simulink library "MotorModelDiscreteTfSL"  (R2016b)
settings: Solver=VariableStepAuto  StartTime=0.0  StopTime=10.0  RelTol=1e-3
undefined symbols (not defined in the file): Z0, Z1, Z2, Znom
settings Model: Creator=oelkawok  LastModifiedBy=oelkawok

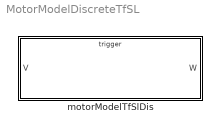
== system MotorModelDiscreteTfSL ==
  motorModelTfSlDis : Subsystem

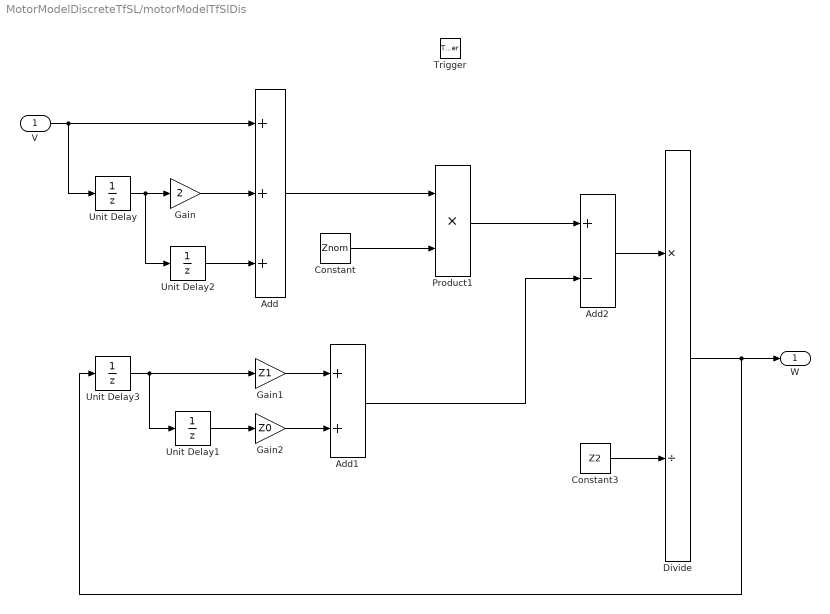
== system MotorModelDiscreteTfSL/motorModelTfSlDis ==
  V : Inport
  Trigger : TriggerPort  TriggerType=function-call  VariantControl=Variant  PortDimensions=1
  Add : Sum  Inputs=+++
  Add1 : Sum
  Add2 : Sum  Inputs=+-
  Constant : Constant  Value=Znom
  Constant3 : Constant  Value=Z2
  Divide : Product  Inputs=*/
  Gain : Gain  Gain=2
  Gain1 : Gain  Gain=Z1
  Gain2 : Gain  Gain=Z0
  Product1 : Product
  Unit Delay{,1..3} (4 alike) : UnitDelay  SampleTime=-1
  W : Outport
  wires:
  V/1 -> Unit Delay/1, Add/1
  Unit Delay/1 -> Unit Delay2/1, Gain/1
  Divide/1 -> W/1, Unit Delay3/1
  Constant/1 -> Product1/2
  Gain/1 -> Add/2
  Unit Delay2/1 -> Add/3
  Add/1 -> Product1/1
  Product1/1 -> Add2/1
  Unit Delay3/1 -> Unit Delay1/1, Gain1/1
  Gain1/1 -> Add1/1
  Unit Delay1/1 -> Gain2/1
  Gain2/1 -> Add1/2
  Add1/1 -> Add2/2
  Add2/1 -> Divide/1
  Constant3/1 -> Divide/2
